simulink model "controller"  (R2024b)
settings: Solver=FixedStepAuto  StartTime=0.0  StopTime=10.0  FixedStep=1/100  RelTol=1e-3
undefined symbols (not defined in the file): MAX_RDB_ENGAGE_SPEED, MAX_TORQUE, MAX_TORQUE_REVERSE, TransmissionState
settings Model: Creator=DAUIN-Win10  LastModifiedBy=Michele
settings OptimizationCC: ReuseModelBlockBuffer=off
settings DebuggingCC: UnconnectedInputMsg=warning  UnconnectedOutputMsg=warning  UnconnectedLineMsg=warning
settings ModelReferenceCC: EnableRefExpFcnMdlSchedulingChecks=on
settings RTWCC: GPUComputeCapability=3.5  DLArmComputeVersion=19.05

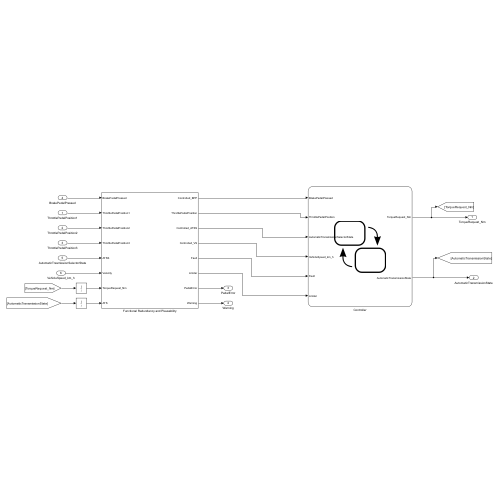
[thumbnail: Simulink's stored preview of the top-level diagram]
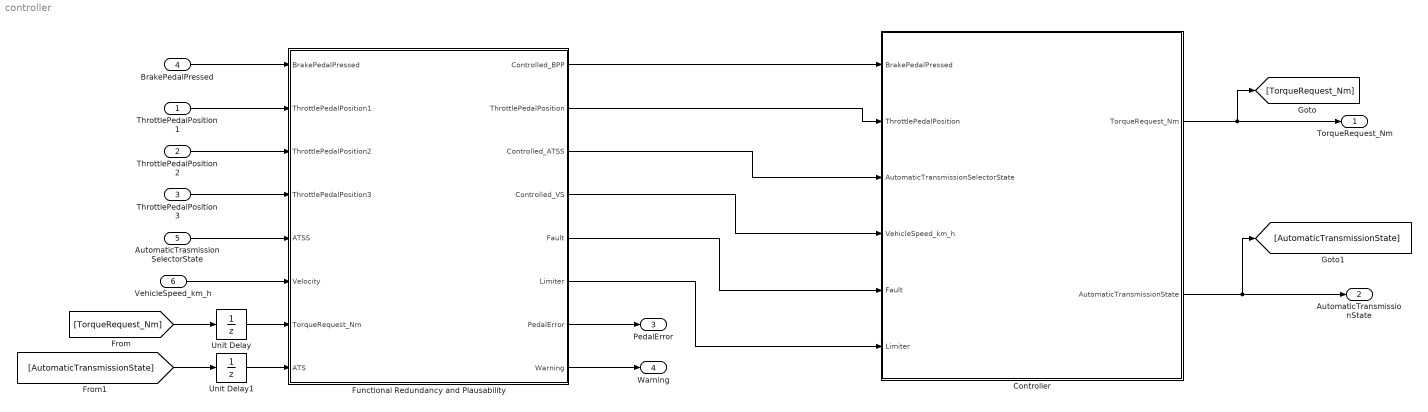
== system controller ==
  ThrottlePedalPosition1 : Inport  OutDataTypeStr=single
  ThrottlePedalPosition2 : Inport  Port=2  OutDataTypeStr=single
  ThrottlePedalPosition3 : Inport  Port=3  OutDataTypeStr=single
  BrakePedalPressed : Inport  Port=4  OutDataTypeStr=boolean
  AutomaticTrasmissionSelectorState : Inport  Port=5  OutDataTypeStr=Enum: TransmissionState
  VehicleSpeed_km_h : Inport  Port=6  OutDataTypeStr=single  Unit=km/h
  Controller : Stateflow chart  TreatAsAtomicUnit=on
      settings: PortSchema="{\"entries\":[{\"content\":{\"sides\":[{\"content\":{\"connectorIds\":[\"In1\",\"In2\",\"In3\",\"In5\",\"In4\",\"In6\"]},\"type\":\"ConnectorPlacement.EquallySpacedRectSide\",\"uuid\":\"8299657d-0502-40c6-b0a0-94f373f4d980\"},{\"content\":{\"connectorIds\":[\"Out1\",\"Out2\"],\"side\":\"RIGHT\"},\"type\":\"ConnectorPlacement.EquallySpacedRectSide\",\"uuid\":\"5efbfe3b-c679-4c7a-ba60-d200927433b8\"},{\"content\":{\"side\":\"TOP\"},\"type\":\"ConnectorPlacement.EquallySpacedRectSide\",\"uuid\":\"8eb3a2db-d3ff-40e0-8198-21b1625c1f86\"}]},\"type\":\"ConnectorPlacement.EquallySpacedConnector\",\"uuid\":\"73ac7723-3127-41a8-b70c-f20bcd517ff0\"}],\"packageUris\":[\"http://schema.mathworks.com/mf0/Connector/R2020b\"],\"version\":\"1.0\"}"
  Functional Redundancy and Plausability : Subsystem
  Unit Delay : UnitDelay  SampleTime=-1  HasFrameUpgradeWarning=on
  Unit Delay1 : UnitDelay  InitialCondition=TransmissionState.Park  SampleTime=-1  HasFrameUpgradeWarning=on
  TorqueRequest_Nm : Outport  OutDataTypeStr=single  Unit=N*m
  AutomaticTransmissionState : Outport  Port=2  OutDataTypeStr=Enum: TransmissionState
  PedalError : Outport  Port=3  OutDataTypeStr=single
  Warning : Outport  Port=4  OutDataTypeStr=Enum: WarningType
  wires:
  Controller/2(AutomaticTransmissionState) -> AutomaticTransmissionState/1, [AutomaticTransmissionState]
  Functional Redundancy and Plausability/2(ThrottlePedalPosition) -> Controller/2(ThrottlePedalPosition)
  ThrottlePedalPosition2/1 -> Functional Redundancy and Plausability/3(ThrottlePedalPosition2)
  Functional Redundancy and Plausability/5(Fault) -> Controller/4(Fault)
  Functional Redundancy and Plausability/7(PedalError) -> PedalError/1
  Controller/1(TorqueRequest_Nm) -> TorqueRequest_Nm/1, [TorqueRequest_Nm]
  BrakePedalPressed/1 -> Functional Redundancy and Plausability/1(BrakePedalPressed)
  Functional Redundancy and Plausability/1(Controlled_BPP) -> Controller/1(BrakePedalPressed)
  Functional Redundancy and Plausability/4(Controlled_VS) -> Controller/5(VehicleSpeed_km_h)
  VehicleSpeed_km_h/1 -> Functional Redundancy and Plausability/6(Velocity)
  Functional Redundancy and Plausability/3(Controlled_ATSS) -> Controller/3(AutomaticTransmissionSelectorState)
  [TorqueRequest_Nm] -> Unit Delay/1
  [AutomaticTransmissionState] -> Unit Delay1/1
  Unit Delay/1 -> Functional Redundancy and Plausability/7(TorqueRequest_Nm)
  Unit Delay1/1 -> Functional Redundancy and Plausability/8(ATS)
  Functional Redundancy and Plausability/6(Limiter) -> Controller/6(Limiter)
  Functional Redundancy and Plausability/8(Warning) -> Warning/1
  AutomaticTrasmissionSelectorState/1 -> Functional Redundancy and Plausability/5(ATSS)
  ThrottlePedalPosition1/1 -> Functional Redundancy and Plausability/2(ThrottlePedalPosition1)
  ThrottlePedalPosition3/1 -> Functional Redundancy and Plausability/4(ThrottlePedalPosition3)

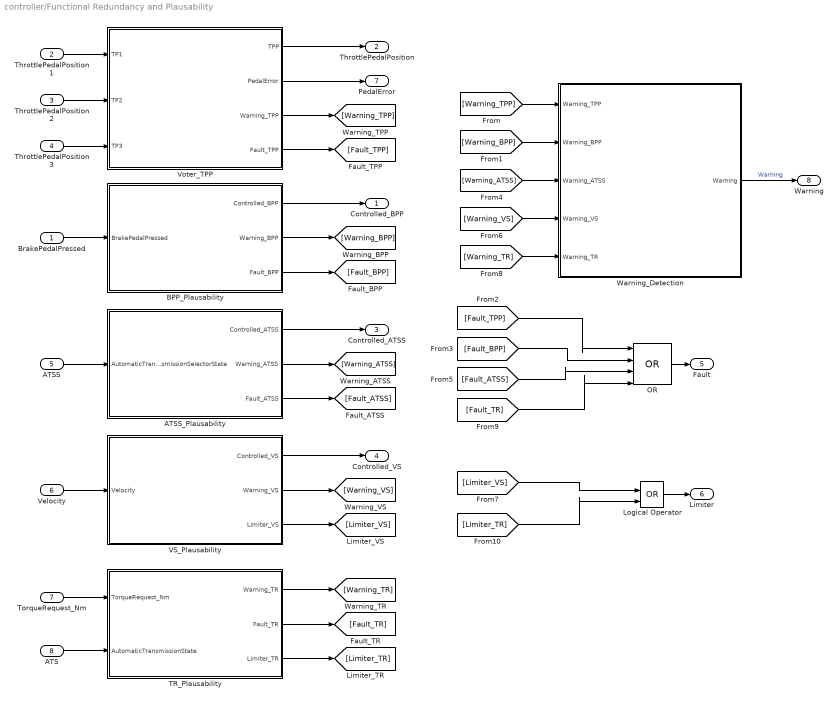
== system controller/Functional Redundancy and Plausability ==
  BrakePedalPressed : Inport
  ThrottlePedalPosition1 : Inport  Port=2
  ThrottlePedalPosition2 : Inport  Port=3
  ThrottlePedalPosition3 : Inport  Port=4
  ATSS : Inport  Port=5  OutDataTypeStr=Enum: TransmissionState
  Velocity : Inport  Port=6  OutDataTypeStr=single
  TorqueRequest_Nm : Inport  Port=7  OutDataTypeStr=single
  ATS : Inport  Port=8  OutDataTypeStr=Enum: TransmissionState
  ATSS_Plausability : MATLAB Function  TreatAsAtomicUnit=on
  BPP_Plausability : MATLAB Function  TreatAsAtomicUnit=on
  Logical Operator : Logic  Operator=OR  IconShape=distinctive  AllPortsSameDT=off  OutDataTypeStr=boolean
  OR : Logic  Operator=OR  Inputs=4  IconShape=distinctive  AllPortsSameDT=off  OutDataTypeStr=boolean
  TR_Plausability : MATLAB Function  TreatAsAtomicUnit=on
  VS_Plausability : MATLAB Function  TreatAsAtomicUnit=on
  Voter_TPP : MATLAB Function  TreatAsAtomicUnit=on
  Warning_Detection : MATLAB Function  TreatAsAtomicUnit=on
  Controlled_BPP : Outport  OutDataTypeStr=boolean
  ThrottlePedalPosition : Outport  Port=2  OutMin=[0]  OutMax=[1]
  Controlled_ATSS : Outport  Port=3  OutDataTypeStr=Enum: TransmissionState
  Controlled_VS : Outport  Port=4  OutDataTypeStr=single
  Fault : Outport  Port=5  OutDataTypeStr=boolean
  Limiter : Outport  Port=6  OutDataTypeStr=boolean
  PedalError : Outport  Port=7  OutDataTypeStr=single
  Warning : Outport  Port=8  OutDataTypeStr=Enum: WarningType
  wires:
  ThrottlePedalPosition1/1 -> Voter_TPP/1(TP1)
  ThrottlePedalPosition2/1 -> Voter_TPP/2(TP2)
  ThrottlePedalPosition3/1 -> Voter_TPP/3(TP3)
  Voter_TPP/1(TPP) -> ThrottlePedalPosition/1
  Voter_TPP/2(PedalError) -> PedalError/1
  BrakePedalPressed/1 -> BPP_Plausability/1(BrakePedalPressed)
  BPP_Plausability/1(Controlled_BPP) -> Controlled_BPP/1
  Velocity/1 -> VS_Plausability/1(Velocity)
  VS_Plausability/1(Controlled_VS) -> Controlled_VS/1
  ATSS/1 -> ATSS_Plausability/1(AutomaticTransmissionSelectorState)
  ATSS_Plausability/1(Controlled_ATSS) -> Controlled_ATSS/1
  TorqueRequest_Nm/1 -> TR_Plausability/1(TorqueRequest_Nm)
  ATS/1 -> TR_Plausability/2(AutomaticTransmissionState)
  OR/1 -> Fault/1
  Voter_TPP/3(Warning_TPP) -> [Warning_TPP]
  BPP_Plausability/2(Warning_BPP) -> [Warning_BPP]
  ATSS_Plausability/2(Warning_ATSS) -> [Warning_ATSS]
  VS_Plausability/2(Warning_VS) -> [Warning_VS]
  TR_Plausability/1(Warning_TR) -> [Warning_TR]
  Voter_TPP/4(Fault_TPP) -> [Fault_TPP]
  BPP_Plausability/3(Fault_BPP) -> [Fault_BPP]
  ATSS_Plausability/3(Fault_ATSS) -> [Fault_ATSS]
  TR_Plausability/2(Fault_TR) -> [Fault_TR]
  VS_Plausability/3(Limiter_VS) -> [Limiter_VS]
  TR_Plausability/3(Limiter_TR) -> [Limiter_TR]
  [Warning_TPP] -> Warning_Detection/1(Warning_TPP)
  [Warning_ATSS] -> Warning_Detection/3(Warning_ATSS)
  [Warning_VS] -> Warning_Detection/4(Warning_VS)
  [Warning_TR] -> Warning_Detection/5(Warning_TR)
  Warning_Detection/1(Warning) -> Warning/1  "Warning"
  [Fault_TPP] -> OR/1
  [Fault_TR] -> OR/4
  [Fault_BPP] -> OR/2
  [Fault_ATSS] -> OR/3
  [Limiter_VS] -> Logical Operator/1
  [Limiter_TR] -> Logical Operator/2
  Logical Operator/1 -> Limiter/1
  [Warning_BPP] -> Warning_Detection/2(Warning_BPP)

== matlab function controller/Functional Redundancy and Plausability/VS_Plausability ==
  data: Velocity input single; Controlled_VS output single; Warning_VS output Enum: WarningType; Limiter_VS output boolean
function [Controlled_VS,Warning_VS,Limiter_VS] = VS_Plausability(Velocity)

Controlled_VS = single(Velocity);
Warning_VS =  WarningType(0);
Limiter_VS = boolean(0);

if (Velocity > 240 || Velocity < -60)

    Warning_VS =  WarningType(1);
    Limiter_VS = boolean(1);

end

== matlab function controller/Functional Redundancy and Plausability/BPP_Plausability ==
  data: BrakePedalPressed input; Controlled_BPP output; Warning_BPP output Enum: WarningType; Fault_BPP output boolean
function [Controlled_BPP,Warning_BPP,Fault_BPP] = BPP_Plausability(BrakePedalPressed)

Warning_BPP = WarningType(0);
Fault_BPP = boolean(0);
Controlled_BPP = boolean(0);

if (BrakePedalPressed == 0 || BrakePedalPressed == 1) 

    Controlled_BPP = boolean(BrakePedalPressed);
        
else

    Warning_BPP = WarningType(2);
    Fault_BPP = boolean(1);

end

== stateflow chart controller/Controller ==
  state Park
    entry:
    AutomaticTransmissionState = TransmissionState.Park;
    during:
    TorqueRequest_Nm = 0;
  state Reverse
    entry:
    AutomaticTransmissionState = TransmissionState.Reverse;
    state BackwardAcceleration
      during:
      TorqueRequest_Nm = -MAX_TORQUE_REVERSE*ThrottlePedalPosition;
    state BackwardRestart
      during:
      TorqueRequest_Nm = -MAX_TORQUE_REVERSE/20;
    state Limiter
      during:
      TorqueRequest_Nm = 0;
    state Stop
      during:
      TorqueRequest_Nm = 0;
    (default) -> BackwardAcceleration
    BackwardRestart -> BackwardAcceleration : [BrakePedalPressed == 0 && ThrottlePedalPosition > 0]
    BackwardAcceleration -> Reverse.Stop [order 1] : [BrakePedalPressed == 1]
    Reverse.Stop -> BackwardAcceleration [order 2] : [BrakePedalPressed == 0]
    (junction 219) -> BackwardAcceleration
    BackwardAcceleration -> (junction 215) [order 2]
    (junction 77) -> BackwardRestart
    (junction 215) -> Reverse.Limiter : [Limiter == 1]
    Reverse.Limiter -> (junction 219) : [Limiter == 0]
    Reverse.Stop -> (junction 77) [order 1] : [BrakePedalPressed == 0 && abs(VehicleSpeed_km_h) <= MAX_RDB_ENGAGE_SPEED]
  state Brake
    entry:
    AutomaticTransmissionState = TransmissionState.Brake;
    state Acceleration
      during:
      TorqueRequest_Nm = MAX_TORQUE*3/2*(ThrottlePedalPosition-1/3);
    state Restart
      during:
      TorqueRequest_Nm = MAX_TORQUE/20;
    state EmergencyStop
      during:
      TorqueRequest_Nm = 0;
    state Stop
      during:
      TorqueRequest_Nm = 0;
    state RegenarativeBraking
      during:
      TorqueRequest_Nm = -MAX_TORQUE*(1-3*ThrottlePedalPosition);
    (default) -> Brake.Acceleration
    Brake.Restart -> Brake.Acceleration [order 2] : [VehicleSpeed_km_h > MAX_RDB_ENGAGE_SPEED]
    Brake.Acceleration -> (junction 123) [order 2] : [BrakePedalPressed == 1 || Limiter == 1]
    (junction 123) -> EmergencyStop
    Brake.Acceleration -> RegenarativeBraking [order 1] : [ThrottlePedalPosition <= 1/3]
    RegenarativeBraking -> Brake.Acceleration [order 1] : [ThrottlePedalPosition > 1/3]
    Brake.Restart -> Brake.Stop [order 1] : [ThrottlePedalPosition <= 1/3 || BrakePedalPressed ==1]
    Brake.Stop -> Brake.Restart [order 1] : [ThrottlePedalPosition > 1/3]
    EmergencyStop -> (junction 127) : [BrakePedalPressed == 0 && Limiter == 0]
    (junction 127) -> RegenarativeBraking
    (junction 134) -> EmergencyStop
    (junction 190) -> EmergencyStop
    RegenarativeBraking -> (junction 134) [order 3] : [BrakePedalPressed == 1]
    Brake.Stop -> (junction 190) [order 2] : [BrakePedalPressed == 1]
    RegenarativeBraking -> Brake.Stop [order 2] : [VehicleSpeed_km_h <= MAX_RDB_ENGAGE_SPEED]
  state Drive
    entry:
    AutomaticTransmissionState = TransmissionState.Drive;
    state Acceleration
      during:
      TorqueRequest_Nm = MAX_TORQUE*ThrottlePedalPosition;
    state Restart
      during:
      TorqueRequest_Nm = MAX_TORQUE/20;
    state Limiter
      during:
      TorqueRequest_Nm = 0;
    state Stop
      during:
      TorqueRequest_Nm = 0;
    (default) -> Drive.Acceleration
    Drive.Restart -> Drive.Acceleration : [BrakePedalPressed == 0 && ThrottlePedalPosition > 0]
    Drive.Acceleration -> Drive.Stop [order 1] : [BrakePedalPressed == 1]
    Drive.Stop -> Drive.Acceleration [order 2] : [BrakePedalPressed == 0]
    (junction 211) -> Drive.Acceleration
    Drive.Acceleration -> (junction 208) [order 2]
    (junction 62) -> Drive.Restart
    (junction 208) -> Drive.Limiter : [Limiter == 1]
    Drive.Limiter -> (junction 211) : [Limiter == 0]
    Drive.Stop -> (junction 62) [order 1] : [BrakePedalPressed == 0 && VehicleSpeed_km_h <= MAX_RDB_ENGAGE_SPEED]
  state Neutral
    entry:
    AutomaticTransmissionState = TransmissionState.Neutral;
    during:
    TorqueRequest_Nm = 0;
  (default) -> Park
  Neutral -> Park [order 3] : [abs(VehicleSpeed_km_h) < 5 && BrakePedalPressed == 1 && AutomaticTransmissionSelectorState == 0 && Fault == 0]
  Park -> Neutral : [BrakePedalPressed == 1 && AutomaticTransmissionSelectorState ~= 0 || Fault == 1]
  Brake -> Drive : [AutomaticTransmissionSelectorState ~= 4 || Fault == 1]
  Drive -> Neutral [order 1] : [AutomaticTransmissionSelectorState == 0 || AutomaticTransmissionSelectorState == 1 || AutomaticTransmissionSelectorState == 2 || Fault == 1]
  Neutral -> Reverse [order 2] : [VehicleSpeed_km_h < 5 && BrakePedalPressed == 1 && AutomaticTransmissionSelectorState == 1 && Fault == 0]
  Reverse -> Neutral : [AutomaticTransmissionSelectorState ~= 1 || Fault == 1]
  Neutral -> Drive [order 1] : [VehicleSpeed_km_h > -5 && BrakePedalPressed == 1 && (AutomaticTransmissionSelectorState == 4|| AutomaticTransmissionSelectorState == 3) && Fault == 0 ]
  Drive -> Brake [order 2] : [ThrottlePedalPosition > 1/3 && AutomaticTransmissionSelectorState == 4 && Fault == 0]
  data: BrakePedalPressed input boolean; ThrottlePedalPosition input single; AutomaticTransmissionSelectorState input Enum: TransmissionState; Fault input boolean; MAX_TORQUE parameter single; MAX_RDB_ENGAGE_SPEED parameter single; TorqueRequest_Nm output single; AutomaticTransmissionState output Enum: TransmissionState; VehicleSpeed_km_h input single; MAX_TORQUE_REVERSE parameter single; Limiter input boolean

== matlab function controller/Functional Redundancy and Plausability/ATSS_Plausability ==
  data: AutomaticTransmissionSelectorState input; Controlled_ATSS output Enum: TransmissionState; Warning_ATSS output Enum: WarningType; Fault_ATSS output
function [Controlled_ATSS,Warning_ATSS,Fault_ATSS] = ATSS_Plausability(AutomaticTransmissionSelectorState)

Controlled_ATSS = TransmissionState(2);
Warning_ATSS = WarningType(0);
Fault_ATSS = boolean(0);

ValidModes = [0 1 2 3 4];

if any(AutomaticTransmissionSelectorState == ValidModes)

    Controlled_ATSS = TransmissionState(AutomaticTransmissionSelectorState);
    
else

    Warning_ATSS = WarningType(2);
    Fault_ATSS = boolean(1);

end

== matlab function controller/Functional Redundancy and Plausability/Voter_TPP ==
  data: TPP output; PedalError output; TP1 input; Warning_TPP output Enum: WarningType; TP2 input; TP3 input; Fault_TPP output
function [TPP,PedalError,Warning_TPP,Fault_TPP] = Voter_TPP(TP1,TP2,TP3)

% Initialization of the output
TPP = single(0);
Warning_TPP = WarningType(0);
PedalError = single(0);
Fault_TPP = boolean(0);
comp = 0.02;

% Comparison between the signals
Diff_1_2 = abs(TP1-TP2);
Diff_1_3 = abs(TP1-TP3);
Diff_2_3 = abs(TP2-TP3);

if (Diff_1_2 <= comp && Diff_1_3 <= comp)

    TPP = (TP1 + TP2 + TP3)/3;
    
elseif Diff_1_2 <= comp

    TPP = (TP1 + TP2)/2;
    Warning_TPP = WarningType(1);
    PedalError = single(3);

elseif Diff_1_3 <= comp

    TPP = (TP1 + TP3)/2;
    Warning_TPP = WarningType(1);
    PedalError = single(2);

elseif Diff_2_3 <= comp

    TPP = (TP2 + TP3)/2;
    Warning_TPP = WarningType(1);
    PedalError = single(1);

else
    
    TPP = single(0);
    Warning_TPP = WarningType(2);
    Fault_TPP = boolean(1);    
    PedalError = single(4);

end

== matlab function controller/Functional Redundancy and Plausability/TR_Plausability ==
  data: Warning_TR output Enum: WarningType; TorqueRequest_Nm input single; Fault_TR output boolean; AutomaticTransmissionState input; Limiter_TR output boolean
function [Warning_TR,Fault_TR,Limiter_TR] = TR_Plausability(TorqueRequest_Nm,AutomaticTransmissionState)

Warning_TR = WarningType(0);
Fault_TR = boolean(0);
Limiter_TR = boolean(0);

PositiveMode = [TransmissionState.Drive, TransmissionState.Brake];
NegativeMode = [TransmissionState.Reverse, TransmissionState.Brake];

if ((TorqueRequest_Nm == 0 ) ...
        || (TorqueRequest_Nm > 0 && any(AutomaticTransmissionState == PositiveMode)) ...
        || (TorqueRequest_Nm < 0  && any(AutomaticTransmissionState == NegativeMode)))
    
    if (TorqueRequest_Nm > 80 || TorqueRequest_Nm < -80 )
        
        Warning_TR =  WarningType(1);
        Limiter_TR = boolean(1);
        
    end

else

    Warning_TR =  WarningType(2);
    Fault_TR = boolean(1); 

end

== matlab function controller/Functional Redundancy and Plausability/Warning_Detection ==
  data: Warning_TPP input Enum: WarningType; Warning output Enum: WarningType; Warning_BPP input Enum: WarningType; Warning_ATSS input Enum: WarningType; Warning_VS input Enum: WarningType; Warning_TR input Enum: WarningType
function Warning = Warning_Detection(Warning_TPP,Warning_BPP,Warning_ATSS,Warning_VS,Warning_TR)

Warning =  WarningType(0);

Warning_set = [Warning_TPP,Warning_BPP,Warning_ATSS,Warning_VS,Warning_TR];

if any(Warning_set ==  WarningType(1))

    Warning =  WarningType(1);

     if any(Warning_set == WarningType(2))
    
        Warning = WarningType(2);
    
     end

elseif any(Warning_set == WarningType(2))

    Warning = WarningType(2);

end
